simulink model "Simulacao"  (Simulink 8.2)
settings: Solver=ode4  SolverMode=SingleTasking  StartTime=0.0  StopTime=20  FixedStep=0.01  RelTol=1e-3
InitFcn:
  | PreLoad;
values from neighbouring files (symbols this model uses):
  A1 = [   0   1 ... (first row only)    [Main.m]    (also in PreLoad.m)
  B1 = [0 ... (first row only)    [PreLoad.m]
  C = [1 0; 0 1]    [PreLoad.m]
  D = zeros(size(C,1), size(B,2))    [PreLoad.m]
  T = 1    [PreLoad.m]
  xk0 = [1.999;0]    [PreLoad.m]
undefined symbols (not defined in the file): A, B, H, R, rho, S, Umax
libraries: simulink x1
settings Model: Creator=Kawakami  LastModifiedBy=Eduardo
settings DataIOCC: LimitDataPoints=off  SaveOutput=off  SaveTime=off  TimeSaveName=t  SignalLoggingName=sigsOut
settings OptimizationCC: BooleanDataType=off
settings DebuggingCC: SaveWithParameterizedLinksMsg=none  SignalResolutionControl=TryResolveAllWithWarning  SolverPrmCheckMsg=none  MultiTaskDSMMsg=warning  MultiTaskCondExecSysMsg=none
settings HardwareCC: TargetUnknown=on
settings RTWCC: IncludeERTFirstTime=on

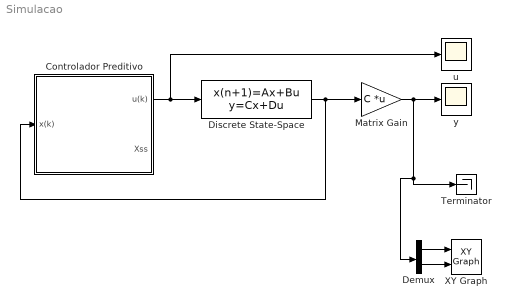
== system Simulacao ==
  "Controlador Preditivo  " : Subsystem  mask{A=A, B=B, H=H, S=S, R=R, Umax=Umax, T=T, rho=rho}
      mask prompts: A "Matriz Agregada A"; B "Matriz Agregada B"; H "H (imagem da Aeq)"; S "S (custo quadrático)"; R "R (custo quadrático)"; Umax "Input Max"; T "T (passo da simulação)"; rho "rho (peso para o Gamma)"
  Demux : Demux  Outputs=2
  Discrete State-Space : DiscreteStateSpace  A=A1  B=B1  C=C  D=D  X0=xk0
  Matrix Gain : Gain  Gain=C  Multiplication=Matrix(K*u)  SaturateOnIntegerOverflow=on  OutDataTypeStr=Inherit: Same as input  ParamDataTypeStr=Inherit: Same as input
  Terminator : Terminator
  XY Graph : simulink/Sinks/XY Graph  xmin=-5  xmax=5  ymin=-5  ymax=5  st=T
  u : Scope
      settings: TimeRange=10  YMin=0.065  YMax=0.1075
  y : Scope
      settings: TimeRange=100  YMin=-191.5000000000001  YMax=48.49999999999989  SaveName=ScopeData2
  wires:
  "Controlador Preditivo  "/1(u(k)) -> Discrete State-Space/1, u/1
  Discrete State-Space/1 -> Matrix Gain/1, "Controlador Preditivo  "/1(x(k))
  Matrix Gain/1 -> Demux/1, Terminator/1, y/1
  Demux/1 -> XY Graph/1
  Demux/2 -> XY Graph/2

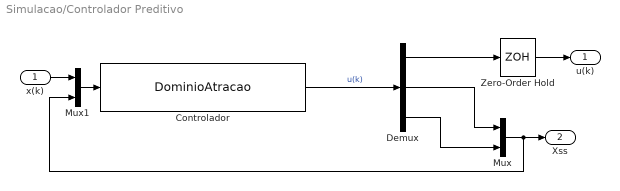
== system Simulacao/Controlador Preditivo   ==
  x(k) : Inport
  Controlador : S-Function  FunctionName=DominioAtracao  Parameters=A, B, S, R, H, Umax, T, rho  EnableBusSupport=off
  Demux : Demux  Outputs=3
  Mux : Mux  Inputs=n
  Mux1 : Mux  Inputs=2
  Zero-Order Hold : ZeroOrderHold  SampleTime=T
  u(k) : Outport
  "Xss " : Outport  Port=2
  wires:
  Zero-Order Hold/1 -> u(k)/1
  Controlador/1 -> Demux/1  "u(k)"
  Demux/1 -> Zero-Order Hold/1
  Demux/2 -> Mux/1
  Mux/1 -> Mux1/2, "Xss "/1
  x(k)/1 -> Mux1/1
  Mux1/1 -> Controlador/1
  Demux/3 -> Mux/2
